simulink model "model_pmxr"  (R2024a)
settings: Solver=VariableStepAuto  StartTime=0.0  StopTime=10.0  RelTol=1e-3
InitFcn:
  | a = 0.672; % M + ma/2 + mb, kg
  | b = 0.0051; % (ma/2 + mb)*L, kg*m
  | % c = 0.0021; % (ma/4 + mb)*L^2 + I, kg*m^2
  | g = 9.81;
  | u = 1;
  | sat = 20;
  | 
  | T1 = 0.2;
  | T2 = 0.1;
  | Tf = 0.05;
  | 
  | x1 = 0;
  | x2 = 0;
  | x3 = 0;
  | x4 = 0;
  | x1p = 0;
  | x2p = 0;
  | x3p = 0;
  | x4p = 0;
  | 
  | r = 1;
  | 
  | b0 = 1;
  | A = [0 1 0;
  |      0 0 1;
  |      0 0 0];
  | b_ = [0; b0; 0];
  | c = [1; 0; 0];
  | 
  | % A_CP = [0 1;
  | %        0 0];
  | %
  | % b_CP = [0; 1];
  | %
  | % w_CL = 70;
  | %
  | % k = place(A_CP', b_CP, -w_CL*[1 1.01])';
  | %
  | % k_ESO = 0.9;
  | %
  | % l = place(A',c,-w_CL*k_ESO*[0.99,1,1.01])';
  | 
  | % k_ESO = 10;
  | 
  | % wc_ = 70;
  | % Kx_ = place(A',b_,-wc_*[1 1])';
  | %
  | % k = [5;5];
  | %
  | % w0 = 60;
  | % l = place(A',c,-w0*[0.99,1,1.01])';
  | 
  | %% Liczenie k
  | w_CL = 5;
  | n=2;
  | k = zeros(n,1);
  | for i = 1:n
  |     k(i) = ((factorial(n))/(factorial(n-i+1)*factorial(i-1)))*w_CL^(n-i+1);
  | end
  | 
  | k_r = [k(2); 1];
  | 
  | %% Liczenie l
  | k_ESO = 50;
  | l = zeros(n+1,1);
  | 
  | for i = 1:n+1
  |     l(i) = (factorial(n+1)/(factorial(n-i+1)*factorial(i)))*(k_ESO)^(i);
  | end
  | 
  | % %% PRZYPISANIE POSZCZEGÓLNYCH L:
  | % l1 = l(1);
  | % l2 = l(2);
  | % %% OKREŚLENIE BETY:
  | % B1 = 3 * k_ESO;
  | % B2 = 3 * k_ESO^2;
  | % B3 = k_ESO^3;
  | 
  | %% W ARTYKULE MADONSKI K,L ODPOWIADA L I B W ARTYKULE JIN H.
  | l1 = k(2);
  | l2 = k(1);
  | 
  | B1 = l(1);
  | B2 = l(2);
  | B3 = l(3);
  | 
  | %% WYZNACZENIE PARAMETRÓW:
  | Kc = (B2 * l2 + B3 * l1)/(b0*(B1 * l1 + B2 + l2));
  | tau_i = (B2 * l2 + B3 * l1)/(B3 * l2);
  | tau_d = (B1 * l2 + B2 * l1 + B3)/(B2 * l2 + B3 * l1);
  | wl = sqrt(B1 * l1 + B2 + l2);
  | zeta_l = (B1 + l1)/(2*sqrt(B1 * l1 + B2 + l2));
  | %% Wzmocnienia regulatora CPID:
  | Kp = Kc;
  | Ki = Kc/tau_i;
  | Kd = Kc * tau_d;
  | 
  | %% NOWE NASTAWY PID
  | % Kp = (k(1)*l(1)+k(2)*l(3))/(b0*(k(2)*l(1)+l(2)+k(1)));
  | % Ki = (k(1)*l(3))/(b0*(k(2)*l(1)+l(2)+k(1)));
  | % Kd = (k(1)*l(1)+k(2)*l(2)+l(3))/(b0*(k(2)*l(1)+l(2)+k(1)));
settings Model: Creator=kubat  LastModifiedBy=kubat

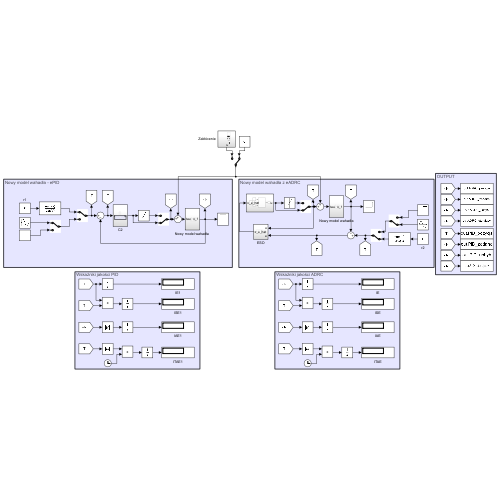
[thumbnail: Simulink's stored preview of the top-level diagram]
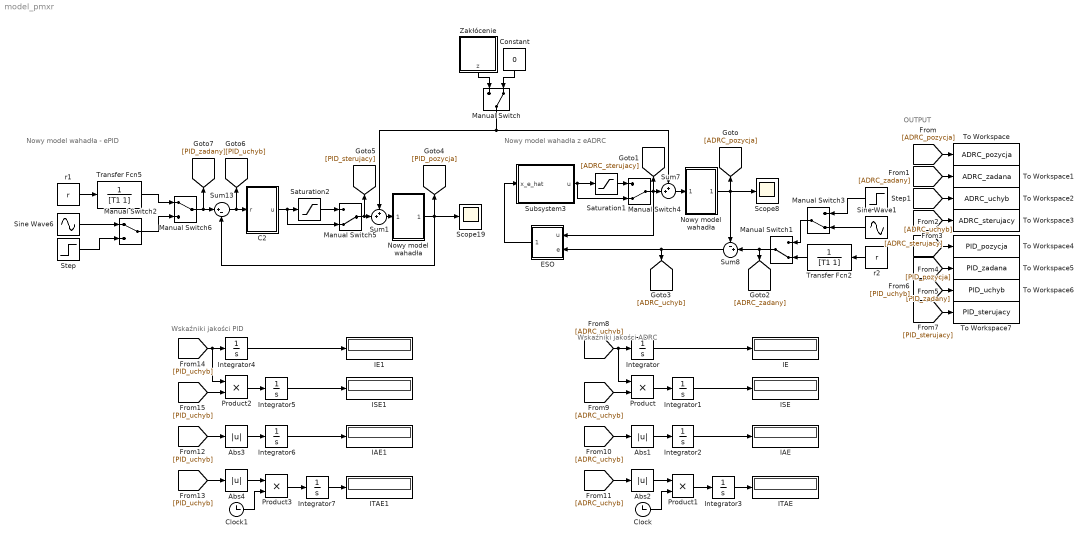
== system model_pmxr ==
  note: OUTPUT
  note: Nowy model wahadła - ePID
  note: Nowy model wahadła z eADRC
  note: Wskaźniki jakości ADRC
  note: Wskaźniki jakości PID
  Abs{1..4} (4 alike) : Abs  SaturateOnIntegerOverflow=off
  C2 : Subsystem
  Clock : Clock
  Clock1 : Clock
  Constant : Constant  Value=0
  ESO : Subsystem
  IAE : Display
  IAE1 : Display
  IE : Display
  IE1 : Display
  ISE : Display
  ISE1 : Display
  ITAE : Display
  ITAE1 : Display
  Integrator{,1..7} (8 alike) : Integrator
  Manual Switch{,1,3..5} (5 alike) : ManualSwitch  CurrentSetting=0
  Manual Switch2 : ManualSwitch
  Manual Switch6 : ManualSwitch
  Nowy model wahadła : Subsystem
  "Nowy model wahadła " : Subsystem
  Product{,1..3} (4 alike) : Product
  Saturation1 : Saturate  UpperLimit=sat  LowerLimit=-sat
  Saturation2 : Saturate  UpperLimit=sat  LowerLimit=-sat
  Scope19 : Scope
  Scope8 : Scope
  Sine Wave1 : Sin  Amplitude=u  SampleTime=0
  Sine Wave6 : Sin  Amplitude=u  SampleTime=0
  Step : Step  After=r  SampleTime=0
  Step1 : Step  After=r  SampleTime=0
  Subsystem3 : Subsystem
  Sum1 : Sum  Inputs=++|
  Sum13 : Sum  Inputs=|+-
  Sum7 : Sum  Inputs=++|
  Sum8 : Sum  Inputs=-+|
  To Workspace : ToWorkspace  VariableName=ADRC_pozycja  SaveFormat=Timeseries  SampleTime=-1
  To Workspace1 : ToWorkspace  VariableName=ADRC_zadana  SaveFormat=Timeseries  SampleTime=-1
  To Workspace2 : ToWorkspace  VariableName=ADRC_uchyb  SaveFormat=Timeseries  SampleTime=-1
  To Workspace3 : ToWorkspace  VariableName=ADRC_sterujacy  SaveFormat=Timeseries  SampleTime=-1
  To Workspace4 : ToWorkspace  VariableName=PID_pozycja  SaveFormat=Timeseries  SampleTime=-1
  To Workspace5 : ToWorkspace  VariableName=PID_zadana  SaveFormat=Timeseries  SampleTime=-1
  To Workspace6 : ToWorkspace  VariableName=PID_uchyb  SaveFormat=Timeseries  SampleTime=-1
  To Workspace7 : ToWorkspace  VariableName=PID_sterujacy  SaveFormat=Timeseries  SampleTime=-1
  Transfer Fcn2 : TransferFcn  Denominator=[T1 1]
  Transfer Fcn5 : TransferFcn  Denominator=[T1 1]
  Zakłócenie : Subsystem
  r1 : Constant  Value=r
  r2 : Constant  Value=r
  wires:
  r2/1 -> Transfer Fcn2/1
  Nowy model wahadła/1(x_1) -> [ADRC_pozycja], Sum8/1, Scope8/1
  r1/1 -> Transfer Fcn5/1
  Transfer Fcn5/1 -> Manual Switch6/1
  Manual Switch6/1 -> [PID_zadany], Sum13/1
  Sum8/1 -> [ADRC_uchyb], ESO/2(e)
  Transfer Fcn2/1 -> Manual Switch1/2
  Manual Switch1/1 -> [ADRC_zadany], Sum8/2
  ESO/1(x_e_hat) -> Subsystem3/1(x_e_hat)
  Manual Switch/1 -> Sum7/1, Sum1/1
  Sum13/1 -> [PID_uchyb], C2/1(r)
  [ADRC_pozycja] -> To Workspace/1
  [ADRC_zadany] -> To Workspace1/1
  [ADRC_uchyb] -> To Workspace2/1
  [ADRC_sterujacy] -> To Workspace3/1
  [PID_sterujacy] -> To Workspace7/1
  [PID_zadany] -> To Workspace5/1
  [PID_pozycja] -> To Workspace4/1
  [PID_uchyb] -> To Workspace6/1
  Constant/1 -> Manual Switch/2
  Zakłócenie/1(z) -> Manual Switch/1
  Clock/1 -> Product1/2
  Integrator3/1 -> ITAE/1
  Abs1/1 -> Integrator2/1
  Integrator2/1 -> IAE/1
  [ADRC_uchyb] -> Abs2/1
  Abs2/1 -> Product1/1
  [ADRC_uchyb] -> Abs1/1
  Integrator/1 -> IE/1
  Product1/1 -> Integrator3/1
  [ADRC_uchyb] -> Product/1, Integrator/1
  Product/1 -> Integrator1/1
  Integrator1/1 -> ISE/1
  [ADRC_uchyb] -> Product/2
  Manual Switch2/1 -> Manual Switch6/2
  Sine Wave6/1 -> Manual Switch2/1
  Step/1 -> Manual Switch2/2
  Sine Wave1/1 -> Manual Switch3/2
  Manual Switch3/1 -> Manual Switch1/1
  Step1/1 -> Manual Switch3/1
  [PID_uchyb] -> Abs4/1
  Abs4/1 -> Product3/1
  [PID_uchyb] -> Abs3/1
  [PID_uchyb] -> Product2/1, Integrator4/1
  Product2/1 -> Integrator5/1
  Clock1/1 -> Product3/2
  Integrator6/1 -> IAE1/1
  Abs3/1 -> Integrator6/1
  Integrator7/1 -> ITAE1/1
  Product3/1 -> Integrator7/1
  [PID_uchyb] -> Product2/2
  Integrator5/1 -> ISE1/1
  Integrator4/1 -> IE1/1
  Sum7/1 -> Nowy model wahadła/1(tau)
  Subsystem3/1(u) -> Manual Switch4/2, Saturation1/1
  Saturation1/1 -> Manual Switch4/1
  Manual Switch4/1 -> ESO/1(u), [ADRC_sterujacy], Sum7/2
  Sum1/1 -> "Nowy model wahadła "/1(tau)
  C2/1(u) -> Manual Switch5/2, Saturation2/1
  Saturation2/1 -> Manual Switch5/1
  Manual Switch5/1 -> [PID_sterujacy], Sum1/2
  "Nowy model wahadła "/1(x_1) -> Scope19/1, Sum13/2, [PID_pozycja]

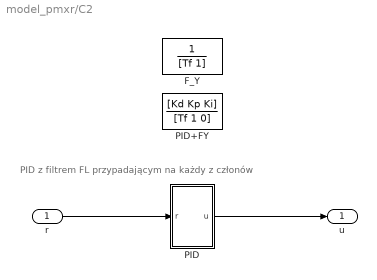
== system model_pmxr/C2 ==
  note: PID z filtrem FL przypadającym na każdy z członów
  r : Inport
  F_Y : TransferFcn  Denominator=[Tf 1]
  PID : Subsystem
  PID+FY : TransferFcn  Numerator=[Kd Kp Ki]  Denominator=[Tf 1 0]
  u : Outport
  wires:
  r/1 -> PID/1(r)
  PID/1(u) -> u/1

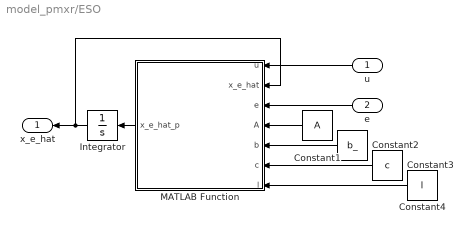
== system model_pmxr/ESO ==
  u : Inport
  e : Inport  Port=2
  Constant1 : Constant  Value=A
  Constant2 : Constant  Value=b_
  Constant3 : Constant  Value=c
  Constant4 : Constant  Value=l
  Integrator : Integrator
  MATLAB Function : MATLAB Function  TreatAsAtomicUnit=on
  x_e_hat : Outport
  wires:
  Constant3/1 -> MATLAB Function/6(c)
  Integrator/1 -> x_e_hat/1, MATLAB Function/2(x_e_hat)
  MATLAB Function/1(x_e_hat_p) -> Integrator/1
  Constant2/1 -> MATLAB Function/5(b)
  e/1 -> MATLAB Function/3(e)
  Constant1/1 -> MATLAB Function/4(A)
  Constant4/1 -> MATLAB Function/7(l)
  u/1 -> MATLAB Function/1(u)

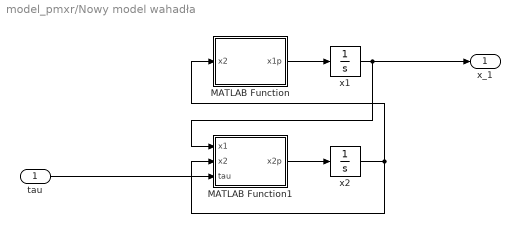
== system model_pmxr/Nowy model wahadła ==
  tau : Inport
  MATLAB Function : MATLAB Function  TreatAsAtomicUnit=on
  MATLAB Function1 : MATLAB Function  TreatAsAtomicUnit=on
  x1 : Integrator
  x2 : Integrator
  x_1 : Outport
  wires:
  x2/1 -> MATLAB Function1/2(x2), MATLAB Function/1(x2)
  x1/1 -> x_1/1, MATLAB Function1/1(x1)
  MATLAB Function/1(x1p) -> x1/1
  tau/1 -> MATLAB Function1/3(tau)
  MATLAB Function1/1(x2p) -> x2/1

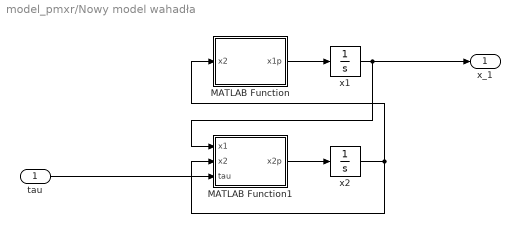
== system model_pmxr/Nowy model wahadła  ==
  tau : Inport
  MATLAB Function : MATLAB Function  TreatAsAtomicUnit=on
  MATLAB Function1 : MATLAB Function  TreatAsAtomicUnit=on
  x1 : Integrator
  x2 : Integrator
  x_1 : Outport
  wires:
  x2/1 -> MATLAB Function1/2(x2), MATLAB Function/1(x2)
  x1/1 -> x_1/1, MATLAB Function1/1(x1)
  MATLAB Function/1(x1p) -> x1/1
  tau/1 -> MATLAB Function1/3(tau)
  MATLAB Function1/1(x2p) -> x2/1

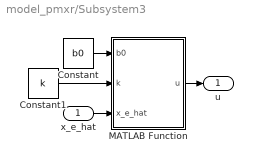
== system model_pmxr/Subsystem3 ==
  x_e_hat : Inport
  Constant : Constant  Value=b0
  Constant1 : Constant  Value=k
  MATLAB Function : MATLAB Function  TreatAsAtomicUnit=on
  u : Outport
  wires:
  Constant/1 -> MATLAB Function/1(b0)
  Constant1/1 -> MATLAB Function/2(k)
  x_e_hat/1 -> MATLAB Function/3(x_e_hat)
  MATLAB Function/1(u) -> u/1

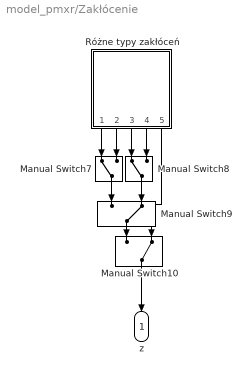
== system model_pmxr/Zakłócenie ==
  Manual Switch10 : ManualSwitch  CurrentSetting=0
  Manual Switch7 : ManualSwitch
  Manual Switch8 : ManualSwitch
  Manual Switch9 : ManualSwitch  CurrentSetting=0
  Różne typy zakłóceń : Subsystem
  z : Outport
  wires:
  Manual Switch10/1 -> z/1
  Manual Switch9/1 -> Manual Switch10/1
  Różne typy zakłóceń/2(Const.2) -> Manual Switch7/2
  Różne typy zakłóceń/5(PWM) -> Manual Switch10/2
  Różne typy zakłóceń/4(nSin.) -> Manual Switch8/2
  Różne typy zakłóceń/1(Const.1) -> Manual Switch7/1
  Manual Switch8/1 -> Manual Switch9/2
  Manual Switch7/1 -> Manual Switch9/1
  Różne typy zakłóceń/3(Sin.1) -> Manual Switch8/1

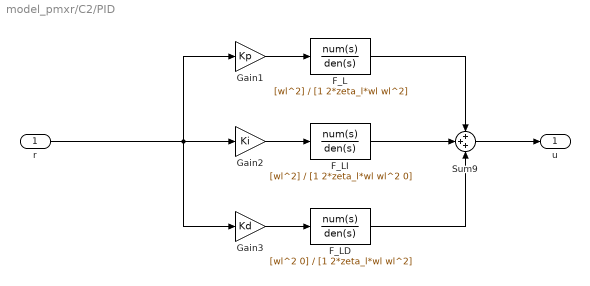
== system model_pmxr/C2/PID ==
  r : Inport
  F_L : TransferFcn  Numerator=[wl^2]  Denominator=[1 2*zeta_l*wl wl^2]
  F_LD : TransferFcn  Numerator=[wl^2 0]  Denominator=[1 2*zeta_l*wl wl^2]
  F_LI : TransferFcn  Numerator=[wl^2]  Denominator=[1 2*zeta_l*wl wl^2 0]
  Gain1 : Gain  Gain=Kp
  Gain2 : Gain  Gain=Ki
  Gain3 : Gain  Gain=Kd
  Sum9 : Sum  Inputs=+++
  u : Outport
  wires:
  Gain1/1 -> F_L/1
  r/1 -> Gain3/1, Gain2/1, Gain1/1
  Sum9/1 -> u/1
  F_L/1 -> Sum9/1
  Gain2/1 -> F_LI/1
  F_LI/1 -> Sum9/2
  Gain3/1 -> F_LD/1
  F_LD/1 -> Sum9/3

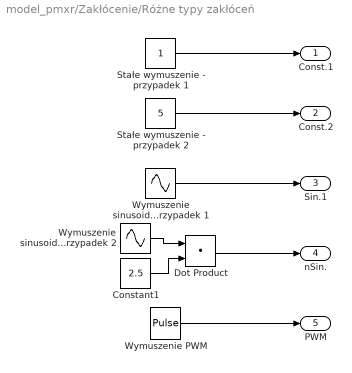
== system model_pmxr/Zakłócenie/Różne typy zakłóceń ==
  Constant1 : Constant  Value=2.5
  Dot Product : DotProduct  OutDataTypeStr=Inherit: Inherit via internal rule
  Stałe wymuszenie - przypadek 1 : Constant
  Stałe wymuszenie - przypadek 2 : Constant  Value=5
  "Wymuszenie PWM " : DiscretePulseGenerator  PulseType=Time based  Period=10  PulseWidth=5
  Wymuszenie sinusoidalne - przypadek 1 : Sin  Amplitude=u  SampleTime=0
  Wymuszenie sinusoidalne - przypadek 2 : Sin  Amplitude=u  SampleTime=0
  Const.1 : Outport
  Const.2 : Outport  Port=2
  Sin.1 : Outport  Port=3
  nSin. : Outport  Port=4
  PWM : Outport  Port=5
  wires:
  Wymuszenie sinusoidalne - przypadek 2/1 -> Dot Product/1
  Constant1/1 -> Dot Product/2
  Stałe wymuszenie - przypadek 1/1 -> Const.1/1
  Wymuszenie sinusoidalne - przypadek 1/1 -> Sin.1/1
  "Wymuszenie PWM "/1 -> PWM/1
  Stałe wymuszenie - przypadek 2/1 -> Const.2/1
  Dot Product/1 -> nSin./1

== matlab function model_pmxr/ESO/MATLAB Function ==
  data: u input; x_e_hat_p output; x_e_hat input; e input; A input; b input; c input; l input
function x_e_hat_p = fcn(u, x_e_hat, e, A, b, c, l)
c = c.';
pom1 = c*x_e_hat;
pom2 = e - pom1;

x_e_hat_p1 = A*x_e_hat-b*u+l*pom2;
x_e_hat_p = x_e_hat_p1(:,1);

== matlab function model_pmxr/Subsystem3/MATLAB Function ==
  data: b0 input; u output; k input; x_e_hat input
function u = fcn(b0, k, x_e_hat)

k = k';
kpom = [k, 1];
b0_1 = 1/b0;
u = b0_1*(kpom*x_e_hat);

== matlab function model_pmxr/Nowy model wahadła/MATLAB Function ==
  data: x2 input; x1p output
function x1p = fcn(x2)

x1p = x2;

== matlab function model_pmxr/Nowy model wahadła/MATLAB Function1 ==
  data: x1 input; x2p output; x2 input; tau input
function x2p = fcn(x1,x2,tau)
%%%PARAMETRY Z ŁAPY JAK COŚ%%%
m = 0.672;
l = 0.5;
g = 9.81;
J = 0.0021;
mi = 0.023;
b = 0.0051;
x2p = 1/(m*l^2+J) * (tau - b*x2 - mi*sign(x2) - l*m*g*cos(x1));

== matlab function model_pmxr/Nowy model wahadła /MATLAB Function ==
  data: x2 input; x1p output
function x1p = fcn(x2)

x1p = x2;

== matlab function model_pmxr/Nowy model wahadła /MATLAB Function1 ==
  data: x1 input; x2p output; x2 input; tau input
function x2p = fcn(x1,x2,tau)
%%%PARAMETRY Z ŁAPY JAK COŚ%%%
m = 0.672;
l = 0.5;
g = 9.81;
J = 0.0021;
mi = 0.023;
b = 0.0051;
x2p = 1/(m*l^2+J) * (tau - b*x2 - mi*sign(x2) - l*m*g*cos(x1));
